simulink model "Spring_OscillationExt2"  (R2017b)
settings: Solver=VariableStepAuto  StartTime=0.0  StopTime=10.0  RelTol=1e-3
values from neighbouring files (symbols this model uses):
  k = k+26    [Caesarcipher.m]
  m = mean(r)    [plotrand.m]
undefined symbols (not defined in the file or in its folder): c
settings Model: Creator=Mahe  LastModifiedBy=Mahe

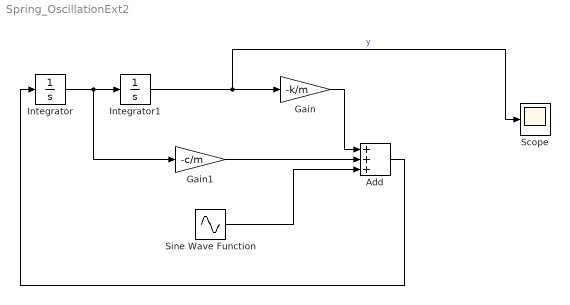
== system Spring_OscillationExt2 ==
  Add : Sum  Inputs=+++
  Gain : Gain  Gain=-k/m
  Gain1 : Gain  Gain=-c/m
  Integrator : Integrator
  Integrator1 : Integrator  InitialCondition=10
  Scope : Scope
  Sine Wave Function : Sin  TimeSource=Use external signal  Amplitude=10  Phase=1.57  SampleTime=0
  wires:
  Add/1 -> Integrator/1
  Gain1/1 -> Add/2
  Integrator/1 -> Gain1/1, Integrator1/1
  Integrator1/1 -> Scope/1, Gain/1  "y"
  Gain/1 -> Add/1
  Sine Wave Function/1 -> Add/3
